simulink model "Equipo04_Sim08_02"  (R2024a)
settings: Solver=VariableStepAuto  StartTime=0.0  StopTime=10.0  RelTol=1e-3
InitFcn:
  | fs = 1e4;
  | Ts = 1/fs;
  | Tb = 0.1;
  | Tc = 0.0125;
  | frameSize = 1000;
libraries: commfilt2 x8, dspsrcs4 x4, commdigbbndpm3 x2, commrandsrc3 x2, commchan3 x1
settings Model: Creator=prust  LastModifiedBy=anita
settings SolverCC: AlgebraicLoopSolver=TrustRegion
settings DataIOCC: ReturnWorkspaceOutputs=off
settings DebuggingCC: UnconnectedInputMsg=warning  UnconnectedOutputMsg=warning  UnconnectedLineMsg=warning  ArithmeticOperatorsInVariantConditions=warning
settings ModelReferenceCC: EnableRefExpFcnMdlSchedulingChecks=on
settings SFSimCC: SimUseLocalCustomCode=off  CustomCodeUndefinedFunction=UseInterfaceOnly
settings RTWCC: RTWUseLocalCustomCode=off  GPUComputeCapability=3.5
settings CodeAppCC: StateflowObjectComments=on

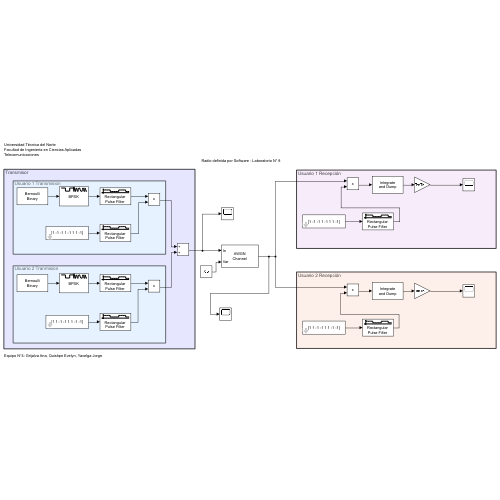
[thumbnail: Simulink's stored preview of the top-level diagram]
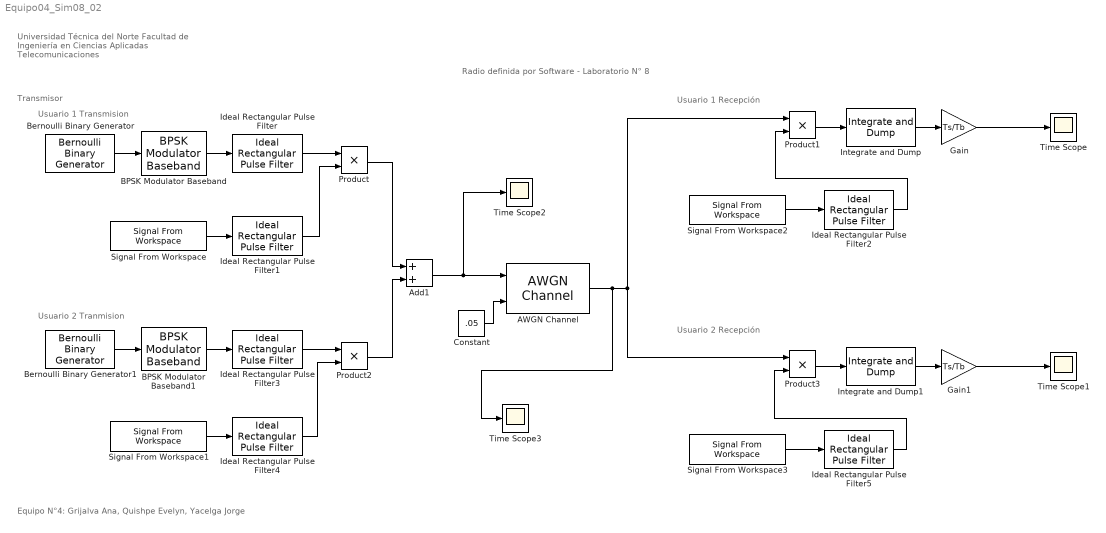
== system Equipo04_Sim08_02 ==
  note: Usuario 1 Recepción
  note: Usuario 1 Transmision
  note: Transmisor
  note: Usuario 2 Tranmision
  note: Usuario 2 Recepción
  note: Universidad Técnica del Norte
      | Facultad de Ingeniería en Ciencias Aplicadas
      | Telecomunicaciones
  note: Radio definida por Software - Laboratorio N° 8
  note: Equipo N°4: Grijalva Ana, Quishpe Evelyn, Yacelga Jorge
  AWGN Channel : commchan3/AWGN Channel  LegacyMode=on  NoiseMethod="Signal to noise ratio  (SNR)"  noiseMode=Variance from port  EbNo=10  EsNo=10  SNR=10  BitsPerSymbol=1  SignalPower=1  SamplesPerSymbol=1  SymbolPeriod=1  VarianceSource=Parameter  Variance=1  RandomStream=Global stream  Seed=67  SimulateUsing=Code generation
  Add1 : Sum
  BPSK Modulator Baseband : commdigbbndpm3/BPSK Modulator Baseband  Ph=0  outDtype=double  outWordLen=16  outUDDataType=sfix(16)  outFracLenMode=Best precision  outFracLen=15  outDataTypeStr=double  outLastDataTypeStr=double
  BPSK Modulator Baseband1 : commdigbbndpm3/BPSK Modulator Baseband  Ph=0  outDtype=double  outWordLen=16  outUDDataType=sfix(16)  outFracLenMode=Best precision  outFracLen=15  outDataTypeStr=double  outLastDataTypeStr=double
  Bernoulli Binary Generator : commrandsrc3/Bernoulli Binary Generator  ProbabilityOfZero=0.5  SeedSource=Auto  Seed=0  SampleTime=Tb  SamplesPerFrame=1  OutputDataType=double  SimulateUsing=Interpreted execution
  Bernoulli Binary Generator1 : commrandsrc3/Bernoulli Binary Generator  ProbabilityOfZero=0.5  SeedSource=Auto  Seed=0  SampleTime=Tb  SamplesPerFrame=1  OutputDataType=double  SimulateUsing=Interpreted execution
  Constant : Constant  Value=.05
  Gain : Gain  Gain=Ts/Tb
  Gain1 : Gain  Gain=Ts/Tb
  Ideal Rectangular Pulse Filter : commfilt2/Ideal Rectangular Pulse Filter  pulseLen=Tb/Ts  pulseDelay=0  InputProcessing=Columns as channels (frame based)  RateOptions=Allow multirate processing  sampMode=Mute  normCheck=off  normMode=Sum of samples  filterGain=1  saveAsFlag=0  roundingMode=Floor  overflowMode=off  firstCoeffDataTypeStr=Inherit: Same word length as input  firstCoeffMin=[]  firstCoeffMax=[]  firstCoeffLastDataTypeStr=Inherit: Same word length as input  outputDataTypeStr=Inherit: Same as accumulator  outputMin=[]  outputMax=[]  outputLastDataTypeStr=Inherit: Same as accumulator
  Ideal Rectangular Pulse Filter{1..2,4..5} (4 alike) : commfilt2/Ideal Rectangular Pulse Filter  pulseLen=Tc/Ts  pulseDelay=0  InputProcessing=Columns as channels (frame based)  RateOptions=Allow multirate processing  sampMode=Mute  normCheck=off  normMode=Sum of samples  filterGain=1  saveAsFlag=0  roundingMode=Floor  overflowMode=off  firstCoeffDataTypeStr=Inherit: Same word length as input  firstCoeffMin=[]  firstCoeffMax=[]  firstCoeffLastDataTypeStr=Inherit: Same word length as input  outputDataTypeStr=Inherit: Same as accumulator  outputMin=[]  outputMax=[]  outputLastDataTypeStr=Inherit: Same as accumulator
  Ideal Rectangular Pulse Filter3 : commfilt2/Ideal Rectangular Pulse Filter  pulseLen=Tb/Ts  pulseDelay=0  InputProcessing=Columns as channels (frame based)  RateOptions=Allow multirate processing  sampMode=Mute  normCheck=off  normMode=Sum of samples  filterGain=1  saveAsFlag=0  roundingMode=Floor  overflowMode=off  firstCoeffDataTypeStr=Inherit: Same word length as input  firstCoeffMin=[]  firstCoeffMax=[]  firstCoeffLastDataTypeStr=Inherit: Same word length as input  outputDataTypeStr=Inherit: Same as accumulator  outputMin=[]  outputMax=[]  outputLastDataTypeStr=Inherit: Same as accumulator
  Integrate and Dump : commfilt2/Integrate and Dump  obssamples=Tb/Ts  offsetsamples=0  nodump=off  roundingMode=Floor  overflowMode=off  outputDataTypeStr=Inherit: Same as accumulator  outputLastDataTypeStr=Inherit: Same as accumulator
  Integrate and Dump1 : commfilt2/Integrate and Dump  obssamples=Tb/Ts  offsetsamples=0  nodump=off  roundingMode=Floor  overflowMode=off  outputDataTypeStr=Inherit: Same as accumulator  outputLastDataTypeStr=Inherit: Same as accumulator
  Product{,1..3} (4 alike) : Product
  Signal From Workspace : dspsrcs4/Signal From Workspace  X=[1 -1 -1 1 -1 1 1 -1]  Ts=Tc  nsamps=1  OutputAfterFinalValue=Cyclic repetition  ignoreOrWarnInputAndFrameLengths=off  OutputFrames=off
  Signal From Workspace1 : dspsrcs4/Signal From Workspace  X=[1 1 -1 -1 1 1 -1 -1]  Ts=Tc  nsamps=1  OutputAfterFinalValue=Cyclic repetition  ignoreOrWarnInputAndFrameLengths=off  OutputFrames=off
  Signal From Workspace2 : dspsrcs4/Signal From Workspace  X=[1 -1 -1 1 -1 1 1 -1]  Ts=Tc  nsamps=1  OutputAfterFinalValue=Cyclic repetition  ignoreOrWarnInputAndFrameLengths=off  OutputFrames=off
  Signal From Workspace3 : dspsrcs4/Signal From Workspace  X=[1 1 -1 -1 1 1 -1 -1]  Ts=Tc  nsamps=1  OutputAfterFinalValue=Cyclic repetition  ignoreOrWarnInputAndFrameLengths=off  OutputFrames=off
  Time Scope{,1..3} (4 alike) : Scope
  wires:
  Bernoulli Binary Generator/1 -> BPSK Modulator Baseband/1
  Ideal Rectangular Pulse Filter/1 -> Product/1
  Signal From Workspace/1 -> Ideal Rectangular Pulse Filter1/1
  Ideal Rectangular Pulse Filter1/1 -> Product/2
  Add1/1 -> Time Scope2/1, AWGN Channel/1
  Constant/1 -> AWGN Channel/2
  Product/1 -> Add1/1
  Signal From Workspace2/1 -> Ideal Rectangular Pulse Filter2/1
  Ideal Rectangular Pulse Filter2/1 -> Product1/2
  AWGN Channel/1 -> Time Scope3/1, Product1/1, Product3/1
  Product1/1 -> Integrate and Dump/1
  Signal From Workspace1/1 -> Ideal Rectangular Pulse Filter4/1
  Ideal Rectangular Pulse Filter4/1 -> Product2/2
  Ideal Rectangular Pulse Filter3/1 -> Product2/1
  Integrate and Dump/1 -> Gain/1
  Product2/1 -> Add1/2
  Bernoulli Binary Generator1/1 -> BPSK Modulator Baseband1/1
  BPSK Modulator Baseband/1 -> Ideal Rectangular Pulse Filter/1
  BPSK Modulator Baseband1/1 -> Ideal Rectangular Pulse Filter3/1
  Gain/1 -> Time Scope/1
  Signal From Workspace3/1 -> Ideal Rectangular Pulse Filter5/1
  Ideal Rectangular Pulse Filter5/1 -> Product3/2
  Product3/1 -> Integrate and Dump1/1
  Integrate and Dump1/1 -> Gain1/1
  Gain1/1 -> Time Scope1/1
